simulink model "RLvali_2021bold"  (R2021b)
settings: Solver=ode15s  StartTime=0.0  StopTime=Tf  FixedStep=0.01  MaxStep=0.05  RelTol=0.5  AbsTol=0.5
model workspace (MATLAB code in the model file):
  | %---------------Critical values---------------%
  | angle_amp = pi/6; % Motor rotate amplitude, ref: pi/4
  | rotateCorrectionCoef = 1.158;
  | criticalFn = 2;
  | 
  | %------values for normalization---------------%
  | % values got by running manual gait
  | rotxNormGain = 1/0.1;
  | rotyNormGain = 1/0.05;
  | rotzNormGain = 1/0.1;
  | 
  | vxNormGain = 1/0.2;
  | vyNormGain = 1/0.2;
  | vzNormGain = 1/0.2;
  | 
  | FnNormGain = 1/15;
  | 
  | %--------values for check done---------------%
  | rotDone = pi/6; % 0.15;
  | legBendDone = pi/3; % actuator max bending angle
  | 
  | 
  | %---------------Robot parameters-------------%
  | % robot size
  | robot_width = 0.15;
  | robot_length = 0.22;
  | 
  | % floor parameters
  | floor_length = 2;
  | floor_width = 2;
  | 
  | % continuum actuator size
  | L_disk = 0.02944;% Disk side length (m)
  | R_w = L_disk/sqrt(3);
  | thickness_disk = 0.004; % Disk thickness (m)
  | thigh_length = 0.06;
  | R_core = 0.005; % Core radius (m)
  | length_core = 0.008; % Core length (m)
  | R_spool = 0.021; % 0.01944; % radius of the spool
  | spool_height = 0.022+0.015;
  | R_pulley = 1e-3;
  | spool_k = 0;
  | spool_d = 0;
  | hole_d = 4e-3;
  | 
  | % Material property
  | rho_PLA = 1.24e3;
  | rho = 1.19e3; % 1.19e3; % Density (kg/m^3)
  | % use rigid joints
  | Pz_stiff = 135000;
  | Pz_damping = 500;
  | S_stiff = 0.0239;
  | S_damping = 7.5e-5;
  | S_low_Bound = -20;
  | S_up_Bound = 20;
  | 
  | R_foot = 0.015; % foot radius (m)
  | 
  | % motor parameter
  | stall_T = 11.2/10; % 11.2 cm*kg, stall torque
  | t_60_deg = 0.2; % 0.09 s
  | V_nomrmal = 6; % corresponding normal voltage
  | Jr = 0.0001; %g*cm^2, robot inertia
  | 
  | % contact force
  | coef_static_friction = 0.315;
  | coef_dynamic_friction = 0.3;
  | crictic_velocity = 0.3; % m/s
  | contact_suf_stiff = 1000; % N/m
  | contact_suf_damp = 50; % N/(m/s)
  | contact_region_width = 2e-3; % m
  | spoolOpacity = 0;
  | tendonColor = [0.902 0.902 0.902];
  | tendonOpacity = 0.1;
  | 
  | % If use point masses
  | MMainFrame = 198; % g
  | MServoMotor = 50.55;
  | MMotorSupport = 12.1;
  | MSpool = 9.2;
  | 
  | % Robot total weight about 2 kg
  | MComposateLoad = 200;
  | 
  | MBuck = 40; % x2
  | MPCB_RPi = 141.3;
  | MLiBattery = 120; % x2
  | MPowerBank = 66.5;
  | isLoadVisible = 0.1;
  | 
  | 
  | MThigh = 26.7963;
  | MCore = 0.747699;
  | MDisk = 1.78642;
  | MFoot = 16.8232;
values from neighbouring files (symbols this model uses):
  N = ceil((A - 8) / (2.285 * abs(Wstop(1) - Wpass(1))))    [testit.m]
  Tf = 10    [longTest.m]    (also in singleTest.m)
  Ts = 0.05    [longTest.m]    (also in singleTest.m)
  x_norm_min = min(x,[],1)    [preprocessData.m]
  x_norm_range = max(x,[],1) - min(x,[],1)    [preprocessData.m]
  y_norm_min = min(y,[],1)    [preprocessData.m]
  y_norm_range = max(y,[],1) - min(y,[],1)    [preprocessData.m]
undefined symbols (not defined in the file or in its folder): alpha_b_gain, alpha_r_gain, DCMotor_K, EntropyList, EntropyWeightList, ExtParts, fnVariance, isCheckDone, isContactBoolean, isUseExtAct, MotorSupport, rotVariance, speedVariance, startAgentTime, TrackStarServo, VRef, WheelCAD, X, Y, Z, z_l_gain
libraries: sm_lib x311, nesl_utility x81, fl_lib x60, ee_lib x24, simulink x16, slpidlib x12, dspstat3 x2, rllib x1
(part 16 of 16)

== system RLvali_2021bold/Robot_body1/RL/Subsystem3/DC servo motor ==
  RefAngle : Inport
  Feedback : Inport  Port=2
  Abs : Abs
  DC Motor : ee_lib/Electromechanical/Brushed Motors/DC Motor  field_option=ee.enum.field_option.pm  Rf=100 Ohm  Lf=1 H  Laf=0.15 H  If0=0 A  parameterization=ee.enum.dcparam_option.torque_speed  Ra=DCMotor_R Ohm  La=9.5 uH  emf_or_torque=ee.enum.emf_or_torque.ki  Kv=7.2e-05 V/rpm  Ki=DCMotor_K N*m/A  T_stall=stall_T N*m  w_max=300 deg/s  w_rated=1.5e+04 rpm  P_rated=0.08 W  V_rated=6 V  lam_param=ee.enum.lam_param.current  i_noload=0.003 A  V_i_noload=6 V  J=0 kg*m^2  lam=DCMotor_Kf N*m/(rad/s)  speed0=0 rpm  enable_fault_armature=simscape.enum.onoff.off  rev_faulted=1 / 3  G_faulted_armature=1e-5 S  fault_trigger_armature=ee.enum.faults.faultTrigger.temporal  t_fault_armature=1 s  max_permissible_current_armature=inf A  t_fail_on_current_armature=1 s  enable_fault_field=simscape.enum.onoff.off  G_faulted_field=1e-5 S  fault_trigger_field=ee.enum.faults.faultTrigger.temporal  t_fault_field=1 s  max_permissible_current_field=inf A  t_fail_on_current_field=1 s  fault_action=simscape.enum.assert.action.none  alpha=3.93e-3 1/K  Tmeas=25 degC  thermal_mass=100 J/K  initial_temperature=25 degC
  Delay : Delay  DelayLength=1
  Electrical Reference2 : fl_lib/Electrical/Electrical Elements/Electrical Reference
  Ideal Angular Velocity Source : fl_lib/Mechanical/Mechanical Sources/Ideal Angular Velocity Source
  Ideal Torque Sensor : fl_lib/Mechanical/Mechanical Sensors/Ideal Torque Sensor
  Mechanical Rotational Reference : fl_lib/Mechanical/Rotational Elements/Mechanical Rotational Reference
  PID Controller : slpidlib/PID Controller  Controller=P  Form=Parallel  TimeDomain=Continuous-time  UseExternalTs=off  SampleTime=-1  IntegratorMethod=Forward Euler  FilterMethod=Forward Euler  ControllerParametersSource=internal  P=24  I=1  D=0  UseFilter=on  N=100  TunerSelectOption=Transfer Function Based (PID Tuner App)  InitialConditionSource=internal  InitialConditionForIntegrator=0  InitialConditionForFilter=0  DifferentiatorICPrevScaledInput=0  ExternalReset=none  TrackingMode=off  Kt=1  LimitOutput=off  SatLimitsSource=internal  UpperSaturationLimit=inf  LowerSaturationLimit=-inf  LinearizeAsGain=on  AntiWindupMode=none  Kb=1  POutMin=[]  POutMax=[]  IOutMin=[]  IOutMax=[]  DOutMin=[]  DOutMax=[]  NOutMin=[]  NOutMax=[]  SumOutMin=[]  SumOutMax=[]  SaturationOutMin=[]  SaturationOutMax=[]  PParamMin=[]  PParamMax=[]  IParamMin=[]  IParamMax=[]  DParamMin=[]  DParamMax=[]  NParamMin=[]  NParamMax=[]  KbParamMin=[]  KbParamMax=[]  KtParamMin=[]  KtParamMax=[]  KbOutMin=[]  KbOutMax=[]  KtOutMin=[]  KtOutMax=[]  IntegratorOutMin=[]  IntegratorOutMax=[]  FilterOutMin=[]  FilterOutMax=[]  SumI1OutMin=[]  SumI1OutMax=[]  SumI2OutMin=[]  SumI2OutMax=[]  SumI3OutMin=[]  SumI3OutMax=[]  SumI4OutMin=[]  SumI4OutMax=[]  SumDOutMin=[]  SumDOutMax=[]  DifferentiatorOutMin=[]  DifferentiatorOutMax=[]  FilterDiffOutCoefMin=[]  FilterDiffOutCoefMax=[]  ReciprocalOutMin=[]  ReciprocalOutMax=[]  SumDenOutMin=[]  SumDenOutMax=[]  SumNumOutMin=[]  SumNumOutMax=[]  DivideOutMin=[]  DivideOutMax=[]  UdiffTsProdOutMin=[]  UdiffTsProdOutMax=[]  NTsProdOutMin=[]  NTsProdOutMax=[]  UintegralTsProdOutMin=[]  UintegralTsProdOutMax=[]  UngainTsProdOutMin=[]  UngainTsProdOutMax=[]  FilterDenConstantOutDataTypeStr=Inherit: Inherit via back propagation  FilterDenConstantOutMin=[]  FilterDenConstantOutMax=[]  PCopyOutDataTypeStr=Inherit: Inherit via back propagation  PCopyOutMin=[]  PCopyOutMax=[]  NCopyOutDataTypeStr=Inherit: Inherit via back propagation  NCopyOutMin=[]  NCopyOutMax=[]  IntegratorContinuousStateAttributes=''  IntegratorStateMustResolveToSignalObject=off  IntegratorRTWStateStorageClass=Auto  FilterContinuousStateAttributes=''  FilterStateMustResolveToSignalObject=off  FilterRTWStateStorageClass=Auto  ParallelPVariant=InternalParameters  IdealPVariant=Disabled  IVariant=Disabled  DVariant=Disabled  IntegratorVariant=Disabled  SatVariant=Disabled  AWVariant=Disabled  PCopyVariant=Disabled  TRVariant=Disabled  FdbkBlocksVariant=Forward  IdealPFdbkVariant=Disabled  SatFdbkVariant=Disabled  DerivativeFilterVariant=Disabled  NVariant=Disabled  NCopyVariant=Disabled_SignalSpec  FilterICVariant=Disabled  IntegratorICVariant=Disabled  ExternalResetVariant=Disabled  TRSumVariant=Passthrough  SumFdbkVariant=Disabled  SumVariant=Passthrough_P  TsampFilterVariant=InternalTs  TsampNgainVariant=Passthrough  TsampIntegralVariant=Disabled_SignalSpec  ExternalSaturationOutDataTypeStr=Inherit: Same as second input
  PS-Simulink Converter : nesl_utility/PS-Simulink Converter  PhysicalDomain=network_engine_domain  SubClassName=ps_output  LeftPortType=input  RightPortType=output  PseudoPeriodic=off  Frequencies=[]  Unit=inherit  AffineConversion=off
      settings: SourceProductBaseCode=PW,SS
  Power Sensor : ee_lib/Sensors & Transducers/Power Sensor  measurement_type=1  averaging_period=1e-4 s
      settings: SourceProductBaseCode=PS
  Simulink to Physical Signal1 : nesl_utility/Simulink-PS Converter  PhysicalDomain=network_engine_domain  SubClassName=ps_input  LeftPortType=input  RightPortType=output  PseudoPeriodic=off  Frequencies=[]  NoiseDistribution=none  NoiseParameters=[]  Unit=V  AffineConversion=off  FilteringAndDerivatives=zero  SimscapeFilterOrder=1  InputFilterTimeConstant=.001  UdotUserProvided=0
      settings: SourceProductBaseCode=PW,SS
  Sum : Sum  Inputs=+-
  Voltage Source : fl_lib/Electrical/Electrical Sources/Controlled Voltage Source
  Torque : PMIOPort  Side=Left
  Speed : PMIOPort  Port=2  Side=Right
  power : Outport
  wires:
  PID Controller/1 -> Simulink to Physical Signal1/1
  RefAngle/1 -> Sum/1
  Feedback/1 -> Sum/2
  Abs/1 -> power/1
  Sum/1 -> PID Controller/1
  PS-Simulink Converter/1 -> Delay/1
  Delay/1 -> Abs/1
  connections:
  DC Motor/RConn1 -- Electrical Reference2/LConn1 -- Voltage Source/RConn2 -- Power Sensor/LConn3
  Ideal Angular Velocity Source/RConn2 -- Mechanical Rotational Reference/LConn1 -- DC Motor/RConn2
  Ideal Torque Sensor/RConn2 -- Torque/RConn1
  Simulink to Physical Signal1/RConn1 -- Voltage Source/RConn1
  DC Motor/LConn2 -- Ideal Torque Sensor/LConn1
  Ideal Angular Velocity Source/RConn1 -- Speed/RConn1
  Ideal Torque Sensor/RConn1 -- Ideal Angular Velocity Source/LConn1
  Voltage Source/LConn1 -- Power Sensor/LConn1
  Power Sensor/LConn2 -- DC Motor/LConn1
  PS-Simulink Converter/LConn1 -- Power Sensor/RConn1

== system RLvali_2021bold/Robot_body1/RR/FR-A/DC servo motor ==
  RefAngle : Inport
  Feedback : Inport  Port=2
  Abs : Abs
  DC Motor : ee_lib/Electromechanical/Brushed Motors/DC Motor  field_option=ee.enum.field_option.pm  Rf=100 Ohm  Lf=1 H  Laf=0.15 H  If0=0 A  parameterization=ee.enum.dcparam_option.torque_speed  Ra=DCMotor_R Ohm  La=9.5 uH  emf_or_torque=ee.enum.emf_or_torque.ki  Kv=7.2e-05 V/rpm  Ki=DCMotor_K N*m/A  T_stall=stall_T N*m  w_max=300 deg/s  w_rated=1.5e+04 rpm  P_rated=0.08 W  V_rated=6 V  lam_param=ee.enum.lam_param.current  i_noload=0.003 A  V_i_noload=6 V  J=0 kg*m^2  lam=DCMotor_Kf N*m/(rad/s)  speed0=0 rpm  enable_fault_armature=simscape.enum.onoff.off  rev_faulted=1 / 3  G_faulted_armature=1e-5 S  fault_trigger_armature=ee.enum.faults.faultTrigger.temporal  t_fault_armature=1 s  max_permissible_current_armature=inf A  t_fail_on_current_armature=1 s  enable_fault_field=simscape.enum.onoff.off  G_faulted_field=1e-5 S  fault_trigger_field=ee.enum.faults.faultTrigger.temporal  t_fault_field=1 s  max_permissible_current_field=inf A  t_fail_on_current_field=1 s  fault_action=simscape.enum.assert.action.none  alpha=3.93e-3 1/K  Tmeas=25 degC  thermal_mass=100 J/K  initial_temperature=25 degC
  Delay : Delay  DelayLength=1
  Electrical Reference2 : fl_lib/Electrical/Electrical Elements/Electrical Reference
  Ideal Angular Velocity Source : fl_lib/Mechanical/Mechanical Sources/Ideal Angular Velocity Source
  Ideal Torque Sensor : fl_lib/Mechanical/Mechanical Sensors/Ideal Torque Sensor
  Mechanical Rotational Reference : fl_lib/Mechanical/Rotational Elements/Mechanical Rotational Reference
  PID Controller : slpidlib/PID Controller  Controller=P  Form=Parallel  TimeDomain=Continuous-time  UseExternalTs=off  SampleTime=-1  IntegratorMethod=Forward Euler  FilterMethod=Forward Euler  ControllerParametersSource=internal  P=24  I=1  D=0  UseFilter=on  N=100  TunerSelectOption=Transfer Function Based (PID Tuner App)  InitialConditionSource=internal  InitialConditionForIntegrator=0  InitialConditionForFilter=0  DifferentiatorICPrevScaledInput=0  ExternalReset=none  TrackingMode=off  Kt=1  LimitOutput=off  SatLimitsSource=internal  UpperSaturationLimit=inf  LowerSaturationLimit=-inf  LinearizeAsGain=on  AntiWindupMode=none  Kb=1  POutMin=[]  POutMax=[]  IOutMin=[]  IOutMax=[]  DOutMin=[]  DOutMax=[]  NOutMin=[]  NOutMax=[]  SumOutMin=[]  SumOutMax=[]  SaturationOutMin=[]  SaturationOutMax=[]  PParamMin=[]  PParamMax=[]  IParamMin=[]  IParamMax=[]  DParamMin=[]  DParamMax=[]  NParamMin=[]  NParamMax=[]  KbParamMin=[]  KbParamMax=[]  KtParamMin=[]  KtParamMax=[]  KbOutMin=[]  KbOutMax=[]  KtOutMin=[]  KtOutMax=[]  IntegratorOutMin=[]  IntegratorOutMax=[]  FilterOutMin=[]  FilterOutMax=[]  SumI1OutMin=[]  SumI1OutMax=[]  SumI2OutMin=[]  SumI2OutMax=[]  SumI3OutMin=[]  SumI3OutMax=[]  SumI4OutMin=[]  SumI4OutMax=[]  SumDOutMin=[]  SumDOutMax=[]  DifferentiatorOutMin=[]  DifferentiatorOutMax=[]  FilterDiffOutCoefMin=[]  FilterDiffOutCoefMax=[]  ReciprocalOutMin=[]  ReciprocalOutMax=[]  SumDenOutMin=[]  SumDenOutMax=[]  SumNumOutMin=[]  SumNumOutMax=[]  DivideOutMin=[]  DivideOutMax=[]  UdiffTsProdOutMin=[]  UdiffTsProdOutMax=[]  NTsProdOutMin=[]  NTsProdOutMax=[]  UintegralTsProdOutMin=[]  UintegralTsProdOutMax=[]  UngainTsProdOutMin=[]  UngainTsProdOutMax=[]  FilterDenConstantOutDataTypeStr=Inherit: Inherit via back propagation  FilterDenConstantOutMin=[]  FilterDenConstantOutMax=[]  PCopyOutDataTypeStr=Inherit: Inherit via back propagation  PCopyOutMin=[]  PCopyOutMax=[]  NCopyOutDataTypeStr=Inherit: Inherit via back propagation  NCopyOutMin=[]  NCopyOutMax=[]  IntegratorContinuousStateAttributes=''  IntegratorStateMustResolveToSignalObject=off  IntegratorRTWStateStorageClass=Auto  FilterContinuousStateAttributes=''  FilterStateMustResolveToSignalObject=off  FilterRTWStateStorageClass=Auto  ParallelPVariant=InternalParameters  IdealPVariant=Disabled  IVariant=Disabled  DVariant=Disabled  IntegratorVariant=Disabled  SatVariant=Disabled  AWVariant=Disabled  PCopyVariant=Disabled  TRVariant=Disabled  FdbkBlocksVariant=Forward  IdealPFdbkVariant=Disabled  SatFdbkVariant=Disabled  DerivativeFilterVariant=Disabled  NVariant=Disabled  NCopyVariant=Disabled_SignalSpec  FilterICVariant=Disabled  IntegratorICVariant=Disabled  ExternalResetVariant=Disabled  TRSumVariant=Passthrough  SumFdbkVariant=Disabled  SumVariant=Passthrough_P  TsampFilterVariant=InternalTs  TsampNgainVariant=Passthrough  TsampIntegralVariant=Disabled_SignalSpec  ExternalSaturationOutDataTypeStr=Inherit: Same as second input
  PS-Simulink Converter : nesl_utility/PS-Simulink Converter  PhysicalDomain=network_engine_domain  SubClassName=ps_output  LeftPortType=input  RightPortType=output  PseudoPeriodic=off  Frequencies=[]  Unit=inherit  AffineConversion=off
      settings: SourceProductBaseCode=PW,SS
  Power Sensor : ee_lib/Sensors & Transducers/Power Sensor  measurement_type=1  averaging_period=1e-4 s
      settings: SourceProductBaseCode=PS
  Simulink to Physical Signal1 : nesl_utility/Simulink-PS Converter  PhysicalDomain=network_engine_domain  SubClassName=ps_input  LeftPortType=input  RightPortType=output  PseudoPeriodic=off  Frequencies=[]  NoiseDistribution=none  NoiseParameters=[]  Unit=V  AffineConversion=off  FilteringAndDerivatives=zero  SimscapeFilterOrder=1  InputFilterTimeConstant=.001  UdotUserProvided=0
      settings: SourceProductBaseCode=PW,SS
  Sum : Sum  Inputs=+-
  Voltage Source : fl_lib/Electrical/Electrical Sources/Controlled Voltage Source
  Torque : PMIOPort  Side=Left
  Speed : PMIOPort  Port=2  Side=Right
  power : Outport
  wires:
  PID Controller/1 -> Simulink to Physical Signal1/1
  RefAngle/1 -> Sum/1
  Feedback/1 -> Sum/2
  Abs/1 -> power/1
  Sum/1 -> PID Controller/1
  PS-Simulink Converter/1 -> Delay/1
  Delay/1 -> Abs/1
  connections:
  DC Motor/RConn1 -- Electrical Reference2/LConn1 -- Voltage Source/RConn2 -- Power Sensor/LConn3
  Ideal Angular Velocity Source/RConn2 -- Mechanical Rotational Reference/LConn1 -- DC Motor/RConn2
  Ideal Torque Sensor/RConn2 -- Torque/RConn1
  Simulink to Physical Signal1/RConn1 -- Voltage Source/RConn1
  DC Motor/LConn2 -- Ideal Torque Sensor/LConn1
  Ideal Angular Velocity Source/RConn1 -- Speed/RConn1
  Ideal Torque Sensor/RConn1 -- Ideal Angular Velocity Source/LConn1
  Voltage Source/LConn1 -- Power Sensor/LConn1
  Power Sensor/LConn2 -- DC Motor/LConn1
  PS-Simulink Converter/LConn1 -- Power Sensor/RConn1

== system RLvali_2021bold/Robot_body1/RR/Subsystem2/DC servo motor ==
  RefAngle : Inport
  Feedback : Inport  Port=2
  Abs : Abs
  DC Motor : ee_lib/Electromechanical/Brushed Motors/DC Motor  field_option=ee.enum.field_option.pm  Rf=100 Ohm  Lf=1 H  Laf=0.15 H  If0=0 A  parameterization=ee.enum.dcparam_option.torque_speed  Ra=DCMotor_R Ohm  La=9.5 uH  emf_or_torque=ee.enum.emf_or_torque.ki  Kv=7.2e-05 V/rpm  Ki=DCMotor_K N*m/A  T_stall=stall_T N*m  w_max=300 deg/s  w_rated=1.5e+04 rpm  P_rated=0.08 W  V_rated=6 V  lam_param=ee.enum.lam_param.current  i_noload=0.003 A  V_i_noload=6 V  J=0 kg*m^2  lam=DCMotor_Kf N*m/(rad/s)  speed0=0 rpm  enable_fault_armature=simscape.enum.onoff.off  rev_faulted=1 / 3  G_faulted_armature=1e-5 S  fault_trigger_armature=ee.enum.faults.faultTrigger.temporal  t_fault_armature=1 s  max_permissible_current_armature=inf A  t_fail_on_current_armature=1 s  enable_fault_field=simscape.enum.onoff.off  G_faulted_field=1e-5 S  fault_trigger_field=ee.enum.faults.faultTrigger.temporal  t_fault_field=1 s  max_permissible_current_field=inf A  t_fail_on_current_field=1 s  fault_action=simscape.enum.assert.action.none  alpha=3.93e-3 1/K  Tmeas=25 degC  thermal_mass=100 J/K  initial_temperature=25 degC
  Delay : Delay  DelayLength=1
  Electrical Reference2 : fl_lib/Electrical/Electrical Elements/Electrical Reference
  Ideal Angular Velocity Source : fl_lib/Mechanical/Mechanical Sources/Ideal Angular Velocity Source
  Ideal Torque Sensor : fl_lib/Mechanical/Mechanical Sensors/Ideal Torque Sensor
  Mechanical Rotational Reference : fl_lib/Mechanical/Rotational Elements/Mechanical Rotational Reference
  PID Controller : slpidlib/PID Controller  Controller=P  Form=Parallel  TimeDomain=Continuous-time  UseExternalTs=off  SampleTime=-1  IntegratorMethod=Forward Euler  FilterMethod=Forward Euler  ControllerParametersSource=internal  P=24  I=1  D=0  UseFilter=on  N=100  TunerSelectOption=Transfer Function Based (PID Tuner App)  InitialConditionSource=internal  InitialConditionForIntegrator=0  InitialConditionForFilter=0  DifferentiatorICPrevScaledInput=0  ExternalReset=none  TrackingMode=off  Kt=1  LimitOutput=off  SatLimitsSource=internal  UpperSaturationLimit=inf  LowerSaturationLimit=-inf  LinearizeAsGain=on  AntiWindupMode=none  Kb=1  POutMin=[]  POutMax=[]  IOutMin=[]  IOutMax=[]  DOutMin=[]  DOutMax=[]  NOutMin=[]  NOutMax=[]  SumOutMin=[]  SumOutMax=[]  SaturationOutMin=[]  SaturationOutMax=[]  PParamMin=[]  PParamMax=[]  IParamMin=[]  IParamMax=[]  DParamMin=[]  DParamMax=[]  NParamMin=[]  NParamMax=[]  KbParamMin=[]  KbParamMax=[]  KtParamMin=[]  KtParamMax=[]  KbOutMin=[]  KbOutMax=[]  KtOutMin=[]  KtOutMax=[]  IntegratorOutMin=[]  IntegratorOutMax=[]  FilterOutMin=[]  FilterOutMax=[]  SumI1OutMin=[]  SumI1OutMax=[]  SumI2OutMin=[]  SumI2OutMax=[]  SumI3OutMin=[]  SumI3OutMax=[]  SumI4OutMin=[]  SumI4OutMax=[]  SumDOutMin=[]  SumDOutMax=[]  DifferentiatorOutMin=[]  DifferentiatorOutMax=[]  FilterDiffOutCoefMin=[]  FilterDiffOutCoefMax=[]  ReciprocalOutMin=[]  ReciprocalOutMax=[]  SumDenOutMin=[]  SumDenOutMax=[]  SumNumOutMin=[]  SumNumOutMax=[]  DivideOutMin=[]  DivideOutMax=[]  UdiffTsProdOutMin=[]  UdiffTsProdOutMax=[]  NTsProdOutMin=[]  NTsProdOutMax=[]  UintegralTsProdOutMin=[]  UintegralTsProdOutMax=[]  UngainTsProdOutMin=[]  UngainTsProdOutMax=[]  FilterDenConstantOutDataTypeStr=Inherit: Inherit via back propagation  FilterDenConstantOutMin=[]  FilterDenConstantOutMax=[]  PCopyOutDataTypeStr=Inherit: Inherit via back propagation  PCopyOutMin=[]  PCopyOutMax=[]  NCopyOutDataTypeStr=Inherit: Inherit via back propagation  NCopyOutMin=[]  NCopyOutMax=[]  IntegratorContinuousStateAttributes=''  IntegratorStateMustResolveToSignalObject=off  IntegratorRTWStateStorageClass=Auto  FilterContinuousStateAttributes=''  FilterStateMustResolveToSignalObject=off  FilterRTWStateStorageClass=Auto  ParallelPVariant=InternalParameters  IdealPVariant=Disabled  IVariant=Disabled  DVariant=Disabled  IntegratorVariant=Disabled  SatVariant=Disabled  AWVariant=Disabled  PCopyVariant=Disabled  TRVariant=Disabled  FdbkBlocksVariant=Forward  IdealPFdbkVariant=Disabled  SatFdbkVariant=Disabled  DerivativeFilterVariant=Disabled  NVariant=Disabled  NCopyVariant=Disabled_SignalSpec  FilterICVariant=Disabled  IntegratorICVariant=Disabled  ExternalResetVariant=Disabled  TRSumVariant=Passthrough  SumFdbkVariant=Disabled  SumVariant=Passthrough_P  TsampFilterVariant=InternalTs  TsampNgainVariant=Passthrough  TsampIntegralVariant=Disabled_SignalSpec  ExternalSaturationOutDataTypeStr=Inherit: Same as second input
  PS-Simulink Converter : nesl_utility/PS-Simulink Converter  PhysicalDomain=network_engine_domain  SubClassName=ps_output  LeftPortType=input  RightPortType=output  PseudoPeriodic=off  Frequencies=[]  Unit=inherit  AffineConversion=off
      settings: SourceProductBaseCode=PW,SS
  Power Sensor : ee_lib/Sensors & Transducers/Power Sensor  measurement_type=1  averaging_period=1e-4 s
      settings: SourceProductBaseCode=PS
  Simulink to Physical Signal1 : nesl_utility/Simulink-PS Converter  PhysicalDomain=network_engine_domain  SubClassName=ps_input  LeftPortType=input  RightPortType=output  PseudoPeriodic=off  Frequencies=[]  NoiseDistribution=none  NoiseParameters=[]  Unit=V  AffineConversion=off  FilteringAndDerivatives=zero  SimscapeFilterOrder=1  InputFilterTimeConstant=.001  UdotUserProvided=0
      settings: SourceProductBaseCode=PW,SS
  Sum : Sum  Inputs=+-
  Voltage Source : fl_lib/Electrical/Electrical Sources/Controlled Voltage Source
  Torque : PMIOPort  Side=Left
  Speed : PMIOPort  Port=2  Side=Right
  power : Outport
  wires:
  PID Controller/1 -> Simulink to Physical Signal1/1
  RefAngle/1 -> Sum/1
  Feedback/1 -> Sum/2
  Abs/1 -> power/1
  Sum/1 -> PID Controller/1
  PS-Simulink Converter/1 -> Delay/1
  Delay/1 -> Abs/1
  connections:
  DC Motor/RConn1 -- Electrical Reference2/LConn1 -- Voltage Source/RConn2 -- Power Sensor/LConn3
  Ideal Angular Velocity Source/RConn2 -- Mechanical Rotational Reference/LConn1 -- DC Motor/RConn2
  Ideal Torque Sensor/RConn2 -- Torque/RConn1
  Simulink to Physical Signal1/RConn1 -- Voltage Source/RConn1
  DC Motor/LConn2 -- Ideal Torque Sensor/LConn1
  Ideal Angular Velocity Source/RConn1 -- Speed/RConn1
  Ideal Torque Sensor/RConn1 -- Ideal Angular Velocity Source/LConn1
  Voltage Source/LConn1 -- Power Sensor/LConn1
  Power Sensor/LConn2 -- DC Motor/LConn1
  PS-Simulink Converter/LConn1 -- Power Sensor/RConn1

== system RLvali_2021bold/Robot_body1/RR/Subsystem3/DC servo motor ==
  RefAngle : Inport
  Feedback : Inport  Port=2
  Abs : Abs
  DC Motor : ee_lib/Electromechanical/Brushed Motors/DC Motor  field_option=ee.enum.field_option.pm  Rf=100 Ohm  Lf=1 H  Laf=0.15 H  If0=0 A  parameterization=ee.enum.dcparam_option.torque_speed  Ra=DCMotor_R Ohm  La=9.5 uH  emf_or_torque=ee.enum.emf_or_torque.ki  Kv=7.2e-05 V/rpm  Ki=DCMotor_K N*m/A  T_stall=stall_T N*m  w_max=300 deg/s  w_rated=1.5e+04 rpm  P_rated=0.08 W  V_rated=6 V  lam_param=ee.enum.lam_param.current  i_noload=0.003 A  V_i_noload=6 V  J=0 kg*m^2  lam=DCMotor_Kf N*m/(rad/s)  speed0=0 rpm  enable_fault_armature=simscape.enum.onoff.off  rev_faulted=1 / 3  G_faulted_armature=1e-5 S  fault_trigger_armature=ee.enum.faults.faultTrigger.temporal  t_fault_armature=1 s  max_permissible_current_armature=inf A  t_fail_on_current_armature=1 s  enable_fault_field=simscape.enum.onoff.off  G_faulted_field=1e-5 S  fault_trigger_field=ee.enum.faults.faultTrigger.temporal  t_fault_field=1 s  max_permissible_current_field=inf A  t_fail_on_current_field=1 s  fault_action=simscape.enum.assert.action.none  alpha=3.93e-3 1/K  Tmeas=25 degC  thermal_mass=100 J/K  initial_temperature=25 degC
  Delay : Delay  DelayLength=1
  Electrical Reference2 : fl_lib/Electrical/Electrical Elements/Electrical Reference
  Ideal Angular Velocity Source : fl_lib/Mechanical/Mechanical Sources/Ideal Angular Velocity Source
  Ideal Torque Sensor : fl_lib/Mechanical/Mechanical Sensors/Ideal Torque Sensor
  Mechanical Rotational Reference : fl_lib/Mechanical/Rotational Elements/Mechanical Rotational Reference
  PID Controller : slpidlib/PID Controller  Controller=P  Form=Parallel  TimeDomain=Continuous-time  UseExternalTs=off  SampleTime=-1  IntegratorMethod=Forward Euler  FilterMethod=Forward Euler  ControllerParametersSource=internal  P=24  I=1  D=0  UseFilter=on  N=100  TunerSelectOption=Transfer Function Based (PID Tuner App)  InitialConditionSource=internal  InitialConditionForIntegrator=0  InitialConditionForFilter=0  DifferentiatorICPrevScaledInput=0  ExternalReset=none  TrackingMode=off  Kt=1  LimitOutput=off  SatLimitsSource=internal  UpperSaturationLimit=inf  LowerSaturationLimit=-inf  LinearizeAsGain=on  AntiWindupMode=none  Kb=1  POutMin=[]  POutMax=[]  IOutMin=[]  IOutMax=[]  DOutMin=[]  DOutMax=[]  NOutMin=[]  NOutMax=[]  SumOutMin=[]  SumOutMax=[]  SaturationOutMin=[]  SaturationOutMax=[]  PParamMin=[]  PParamMax=[]  IParamMin=[]  IParamMax=[]  DParamMin=[]  DParamMax=[]  NParamMin=[]  NParamMax=[]  KbParamMin=[]  KbParamMax=[]  KtParamMin=[]  KtParamMax=[]  KbOutMin=[]  KbOutMax=[]  KtOutMin=[]  KtOutMax=[]  IntegratorOutMin=[]  IntegratorOutMax=[]  FilterOutMin=[]  FilterOutMax=[]  SumI1OutMin=[]  SumI1OutMax=[]  SumI2OutMin=[]  SumI2OutMax=[]  SumI3OutMin=[]  SumI3OutMax=[]  SumI4OutMin=[]  SumI4OutMax=[]  SumDOutMin=[]  SumDOutMax=[]  DifferentiatorOutMin=[]  DifferentiatorOutMax=[]  FilterDiffOutCoefMin=[]  FilterDiffOutCoefMax=[]  ReciprocalOutMin=[]  ReciprocalOutMax=[]  SumDenOutMin=[]  SumDenOutMax=[]  SumNumOutMin=[]  SumNumOutMax=[]  DivideOutMin=[]  DivideOutMax=[]  UdiffTsProdOutMin=[]  UdiffTsProdOutMax=[]  NTsProdOutMin=[]  NTsProdOutMax=[]  UintegralTsProdOutMin=[]  UintegralTsProdOutMax=[]  UngainTsProdOutMin=[]  UngainTsProdOutMax=[]  FilterDenConstantOutDataTypeStr=Inherit: Inherit via back propagation  FilterDenConstantOutMin=[]  FilterDenConstantOutMax=[]  PCopyOutDataTypeStr=Inherit: Inherit via back propagation  PCopyOutMin=[]  PCopyOutMax=[]  NCopyOutDataTypeStr=Inherit: Inherit via back propagation  NCopyOutMin=[]  NCopyOutMax=[]  IntegratorContinuousStateAttributes=''  IntegratorStateMustResolveToSignalObject=off  IntegratorRTWStateStorageClass=Auto  FilterContinuousStateAttributes=''  FilterStateMustResolveToSignalObject=off  FilterRTWStateStorageClass=Auto  ParallelPVariant=InternalParameters  IdealPVariant=Disabled  IVariant=Disabled  DVariant=Disabled  IntegratorVariant=Disabled  SatVariant=Disabled  AWVariant=Disabled  PCopyVariant=Disabled  TRVariant=Disabled  FdbkBlocksVariant=Forward  IdealPFdbkVariant=Disabled  SatFdbkVariant=Disabled  DerivativeFilterVariant=Disabled  NVariant=Disabled  NCopyVariant=Disabled_SignalSpec  FilterICVariant=Disabled  IntegratorICVariant=Disabled  ExternalResetVariant=Disabled  TRSumVariant=Passthrough  SumFdbkVariant=Disabled  SumVariant=Passthrough_P  TsampFilterVariant=InternalTs  TsampNgainVariant=Passthrough  TsampIntegralVariant=Disabled_SignalSpec  ExternalSaturationOutDataTypeStr=Inherit: Same as second input
  PS-Simulink Converter : nesl_utility/PS-Simulink Converter  PhysicalDomain=network_engine_domain  SubClassName=ps_output  LeftPortType=input  RightPortType=output  PseudoPeriodic=off  Frequencies=[]  Unit=inherit  AffineConversion=off
      settings: SourceProductBaseCode=PW,SS
  Power Sensor : ee_lib/Sensors & Transducers/Power Sensor  measurement_type=1  averaging_period=1e-4 s
      settings: SourceProductBaseCode=PS
  Simulink to Physical Signal1 : nesl_utility/Simulink-PS Converter  PhysicalDomain=network_engine_domain  SubClassName=ps_input  LeftPortType=input  RightPortType=output  PseudoPeriodic=off  Frequencies=[]  NoiseDistribution=none  NoiseParameters=[]  Unit=V  AffineConversion=off  FilteringAndDerivatives=zero  SimscapeFilterOrder=1  InputFilterTimeConstant=.001  UdotUserProvided=0
      settings: SourceProductBaseCode=PW,SS
  Sum : Sum  Inputs=+-
  Voltage Source : fl_lib/Electrical/Electrical Sources/Controlled Voltage Source
  Torque : PMIOPort  Side=Left
  Speed : PMIOPort  Port=2  Side=Right
  power : Outport
  wires:
  PID Controller/1 -> Simulink to Physical Signal1/1
  RefAngle/1 -> Sum/1
  Feedback/1 -> Sum/2
  Abs/1 -> power/1
  Sum/1 -> PID Controller/1
  PS-Simulink Converter/1 -> Delay/1
  Delay/1 -> Abs/1
  connections:
  DC Motor/RConn1 -- Electrical Reference2/LConn1 -- Voltage Source/RConn2 -- Power Sensor/LConn3
  Ideal Angular Velocity Source/RConn2 -- Mechanical Rotational Reference/LConn1 -- DC Motor/RConn2
  Ideal Torque Sensor/RConn2 -- Torque/RConn1
  Simulink to Physical Signal1/RConn1 -- Voltage Source/RConn1
  DC Motor/LConn2 -- Ideal Torque Sensor/LConn1
  Ideal Angular Velocity Source/RConn1 -- Speed/RConn1
  Ideal Torque Sensor/RConn1 -- Ideal Angular Velocity Source/LConn1
  Voltage Source/LConn1 -- Power Sensor/LConn1
  Power Sensor/LConn2 -- DC Motor/LConn1
  PS-Simulink Converter/LConn1 -- Power Sensor/RConn1

== matlab function RLvali_2021bold/Sensors1/q2r ==
  data: u input; y output
function y = fcn(u)


% The input is the quaternion and the output is the rotational angle in
% X,Y,Z axis in radius
y = flip(euler(quaternion(u(1),u(2),u(3),u(4)),'ZYX','point'))';

== matlab function RLvali_2021bold/Extropy/MATLAB Function ==
  data: EntropyWeightList input; EntropyList input; isDone input
function fcn(EntropyWeightList, EntropyList, isDone)
    coder.extrinsic('assignin', 'currentTimestr', 'now', 'evalin', 'datestr');
    if isDone
        xlimEntropy = find(EntropyWeightList,1,'Last')-1;

        figure(5);
        set(gcf,'Visible','on')

        subplot(2,1,1)
        plot(EntropyList(2:end))
        xlabel('Samples')
        ylabel('Expected Entropy')
        xlim([-0.1,xlimEntropy])

        subplot(2,1,2)
        plot(EntropyWeightList(2:end))
        xlabel('Samples')
        ylabel('Entropy Weight')
        xlim([-0.1,xlimEntropy])
        % hold off

        % save the collected data
        evalin('base', 'currentTimestr = datestr(now,''yyyy_mmmm_dd_HH_MM'');');
        evalin('base', 'data.obsv = obsv_vec;');
        evalin('base', 'data.act = act_vec;');
        evalin('base', 'save(append(''Entropy\Entropy_'', currentTimestr,''.mat''), ''data'');');
    end
end

== matlab function RLvali_2021bold/Extropy/MATLAB Function1 ==
  settings: updateMethod=DISCRETE  sampleTime=Ts
  data: time input; obsv input; act input
function store_data(time, obsv, act)
    coder.extrinsic('assignin', 'evalin');
    if time == 0
        assignin("base", "obsv_vec", [ones(1, 10); zeros(100, 10)]);
        assignin("base", "act_vec", [ones(1, 4); zeros(100, 4)]);
        evalin('base', 'clear(''data'');');
    end

    assignin("base", "obsv", obsv');
    assignin("base", "act", act');
    evalin('base', '[rows, ~] = find(obsv_vec, 1, ''last'');');
    evalin('base', 'obsv_vec(rows + 1, :) = obsv;');
    evalin('base', 'act_vec(rows + 1, :) = act;');

== matlab function RLvali_2021bold/Act2Angle/Subsystem2/MATLAB Function ==
  data: alpha_r input; alpha_A output; alpha_b input; z_l input; alpha_B output; alpha_C output
function [alpha_A, alpha_B, alpha_C]= fcn(alpha_r, alpha_b, z_l)

L_disk = 0.02944;% Disk side length (m)
R_spool = 0.021;
R_w = L_disk/sqrt(3);

alpha_A = (-R_w*alpha_b*cos(-alpha_r)+z_l)/R_spool;
alpha_B = (-R_w*alpha_b*cos(-alpha_r+2*pi/3)+z_l)/R_spool;
alpha_C = (-R_w*alpha_b*cos(-alpha_r+4*pi/3)+z_l)/R_spool;

== matlab function RLvali_2021bold/Act2Angle/Subsystem2/MATLAB Function1 ==
  data: alpha_r input; alpha_A output; alpha_b input; z_l input; alpha_B output; alpha_C output
function [alpha_A, alpha_B, alpha_C]= fcn(alpha_r, alpha_b, z_l)

L_disk = 0.02944;% Disk side length (m)
R_spool = 0.021;
R_w = L_disk/sqrt(3);

alpha_A = (-R_w*alpha_b*cos(-alpha_r)+z_l)/R_spool;
alpha_B = (-R_w*alpha_b*cos(-alpha_r+2*pi/3)+z_l)/R_spool;
alpha_C = (-R_w*alpha_b*cos(-alpha_r+4*pi/3)+z_l)/R_spool;

== matlab function RLvali_2021bold/Robot_body1/sensFL/q2r ==
  data: u input; y output
function y = fcn(u)


% The input is the quaternion and the output is the rotational angle in
% X,Y,Z axis in radius
y = flip(euler(quaternion(u(1),u(2),u(3),u(4)),'ZYX','point'))';

== matlab function RLvali_2021bold/Robot_body1/sensFR/q2r ==
  data: u input; y output
function y = fcn(u)


% The input is the quaternion and the output is the rotational angle in
% X,Y,Z axis in radius
y = flip(euler(quaternion(u(1),u(2),u(3),u(4)),'ZYX','point'))';

== matlab function RLvali_2021bold/Act2Angle/Subsystem1/MATLAB Function ==
  data: alpha_r input; alpha_A output; alpha_b input; z_l input; alpha_B output; alpha_C output
function [alpha_A, alpha_B, alpha_C]= fcn(alpha_r, alpha_b, z_l)

L_disk = 0.02944;% Disk side length (m)
R_spool = 0.021;
R_w = L_disk/sqrt(3);

alpha_A = (-R_w*alpha_b*cos(-alpha_r)+z_l)/R_spool;
alpha_B = (-R_w*alpha_b*cos(-alpha_r+2*pi/3)+z_l)/R_spool;
alpha_C = (-R_w*alpha_b*cos(-alpha_r+4*pi/3)+z_l)/R_spool;

== matlab function RLvali_2021bold/Robot_body1/sensRL/q2r ==
  data: u input; y output
function y = fcn(u)


% The input is the quaternion and the output is the rotational angle in
% X,Y,Z axis in radius
y = flip(euler(quaternion(u(1),u(2),u(3),u(4)),'ZYX','point'))';

== matlab function RLvali_2021bold/Act2Angle/Subsystem1/MATLAB Function1 ==
  data: alpha_r input; alpha_A output; alpha_b input; z_l input; alpha_B output; alpha_C output
function [alpha_A, alpha_B, alpha_C]= fcn(alpha_r, alpha_b, z_l)

L_disk = 0.02944;% Disk side length (m)
R_spool = 0.021;
R_w = L_disk/sqrt(3);

alpha_A = (-R_w*alpha_b*cos(-alpha_r)+z_l)/R_spool;
alpha_B = (-R_w*alpha_b*cos(-alpha_r+2*pi/3)+z_l)/R_spool;
alpha_C = (-R_w*alpha_b*cos(-alpha_r+4*pi/3)+z_l)/R_spool;

== matlab function RLvali_2021bold/Robot_body1/sensRR/q2r ==
  data: u input; y output
function y = fcn(u)


% The input is the quaternion and the output is the rotational angle in
% X,Y,Z axis in radius
y = flip(euler(quaternion(u(1),u(2),u(3),u(4)),'ZYX','point'))';
